simulink model "tarea3Sim2"  (R2022b)
settings: Solver=VariableStepAuto  StartTime=0.0  StopTime=60  RelTol=1e-3
undefined symbols (not defined in the file): ModelMRAC, ModelReference, Ts
settings Model: Creator=felip  LastModifiedBy=felip

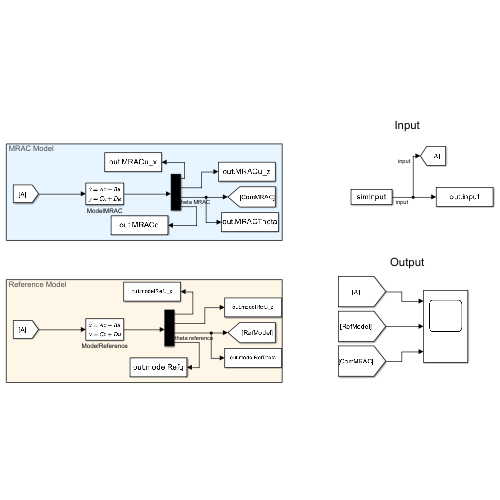
[thumbnail: Simulink's stored preview of the top-level diagram]
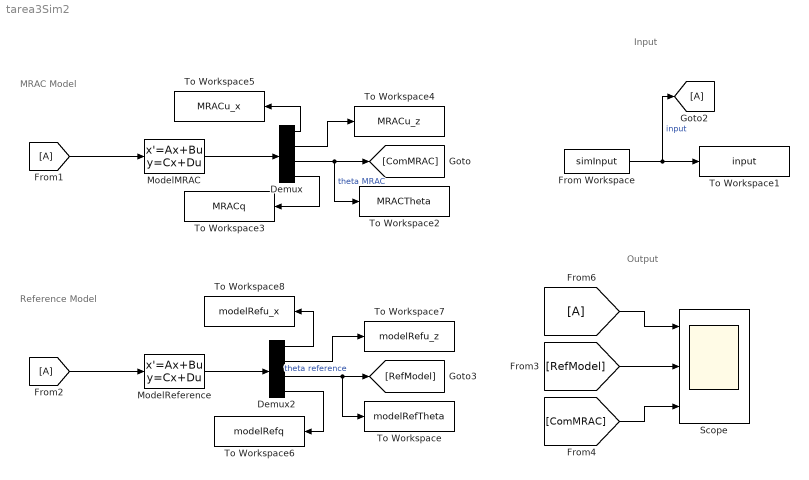
== system tarea3Sim2 ==
  note: Input
  note: MRAC Model
  note: Reference Model
  note: Output
  Demux : Demux
  Demux2 : Demux
  From Workspace : FromWorkspace  VariableName=simInput  SampleTime=Ts
  From1 : From
  From2 : From
  From6 : From
  Goto2 : Goto
  ModelMRAC : StateSpace  A=ModelMRAC.A  B=ModelMRAC.B  C=ModelMRAC.C  D=ModelMRAC.D  InitialCondition=0  ParameterTunability=Unconstrained
  ModelReference : StateSpace  A=ModelReference.A  B=ModelReference.B  C=ModelReference.C  D=ModelReference.D  InitialCondition=0  ParameterTunability=Unconstrained
  Scope : Scope  NumInputPorts=3
  To Workspace : ToWorkspace  VariableName=modelRefTheta  SaveFormat=Timeseries  SampleTime=-1
  To Workspace1 : ToWorkspace  VariableName=input  SaveFormat=Timeseries  SampleTime=Ts
  To Workspace2 : ToWorkspace  VariableName=MRACTheta  SaveFormat=Timeseries  SampleTime=-1
  To Workspace3 : ToWorkspace  VariableName=MRACq  SaveFormat=Timeseries  SampleTime=-1
  To Workspace4 : ToWorkspace  VariableName=MRACu_z  SaveFormat=Timeseries  SampleTime=-1
  To Workspace5 : ToWorkspace  VariableName=MRACu_x  SaveFormat=Timeseries  SampleTime=-1
  To Workspace6 : ToWorkspace  VariableName=modelRefq  SaveFormat=Timeseries  SampleTime=-1
  To Workspace7 : ToWorkspace  VariableName=modelRefu_z  SaveFormat=Timeseries  SampleTime=-1
  To Workspace8 : ToWorkspace  VariableName=modelRefu_x  SaveFormat=Timeseries  SampleTime=-1
  wires:
  From1/1 -> ModelMRAC/1
  ModelMRAC/1 -> Demux/1
  Demux/3 -> [ComMRAC], To Workspace2/1  "theta MRAC"
  Demux2/3 -> [RefModel], To Workspace/1  "theta reference"
  From2/1 -> ModelReference/1
  ModelReference/1 -> Demux2/1
  [RefModel] -> Scope/2
  [ComMRAC] -> Scope/3
  From6/1 -> Scope/1
  Demux2/2 -> To Workspace7/1
  Demux2/1 -> To Workspace8/1
  Demux/4 -> To Workspace3/1
  Demux/2 -> To Workspace4/1
  Demux/1 -> To Workspace5/1
  Demux2/4 -> To Workspace6/1
  From Workspace/1 -> Goto2/1, To Workspace1/1  "input"
